simulink model "T02_SimModel_02"  (R2016b)
settings: Solver=ode1  StartTime=0.0002  StopTime=2000  FixedStep=0.01  RelTol=1e-3
libraries: simulink x1
settings Model: Creator=Maksim  LastModifiedBy=Maksim

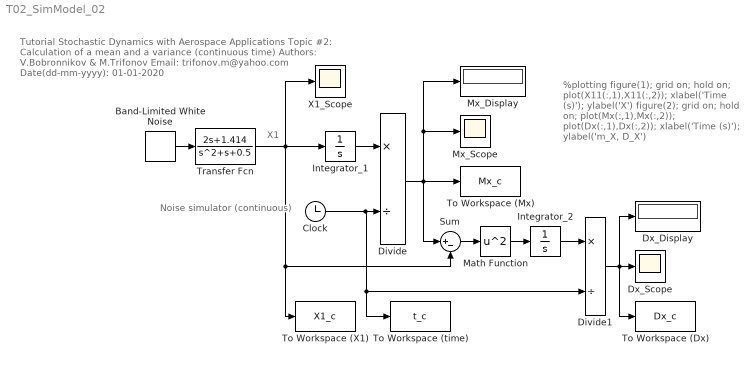
== system T02_SimModel_02 ==
  note: %plotting
      | figure(1); grid on; hold on;
      | plot(X11(:,1),X11(:,2));
      | xlabel('Time (s)'); ylabel('X')
      | figure(2); grid on; hold on;
      | plot(Mx(:,1),Mx(:,2));
      | plot(Dx(:,1),Dx(:,2));
      | xlabel('Time (s)'); ylabel('m_X, D_X')
  note: X1
  note: Noise simulator
      | (continuous)
  note: Tutorial Stochastic Dynamics with Aerospace Applications
      | Topic #2: Calculation of a mean and a variance (continuous time)
      | Authors: V.Bobronnikov & M.Trifonov
      | Email: trifonov.m@yahoo.com
      | Date(dd-mm-yyyy): 01-01-2020
  Band-Limited White Noise : simulink/Sources/Band-Limited White Noise  Cov=[1]  Ts=0.01  seed=[23346]
  Clock : Clock
  Divide : Product  Inputs=*/
  Divide1 : Product  Inputs=*/
  Dx_Display : Display
  Dx_Scope : Scope
  Integrator_1 : Integrator
  Integrator_2 : Integrator
  Math Function : Math  Operator=square  SaturateOnIntegerOverflow=on
  Mx_Display : Display
  Mx_Scope : Scope
  Sum : Sum  Inputs=|+-
  To Workspace (Dx) : ToWorkspace  VariableName=Dx_c  SampleTime=-1
  To Workspace (Mx) : ToWorkspace  VariableName=Mx_c  SampleTime=-1
  To Workspace (X1) : ToWorkspace  VariableName=X1_c  SampleTime=-1
  To Workspace (time) : ToWorkspace  VariableName=t_c  SampleTime=-1
  Transfer Fcn : TransferFcn  Numerator=[2 1.414]  Denominator=[1 1 0.5]
  X1_Scope : Scope
  wires:
  Band-Limited White Noise/1 -> Transfer Fcn/1
  Transfer Fcn/1 -> X1_Scope/1, To Workspace (X1)/1, Sum/2, Integrator_1/1
  Integrator_1/1 -> Divide/1
  Clock/1 -> To Workspace (time)/1, Divide1/2, Divide/2
  Divide/1 -> To Workspace (Mx)/1, Mx_Display/1, Mx_Scope/1, Sum/1
  Sum/1 -> Math Function/1
  Math Function/1 -> Integrator_2/1
  Integrator_2/1 -> Divide1/1
  Divide1/1 -> To Workspace (Dx)/1, Dx_Scope/1, Dx_Display/1
